simulink model "rhomodel"  (R2020a)
settings: Solver=VariableStepAuto  StartTime=0.0  StopTime=10.0  RelTol=1e-3
settings Model: Creator=marce  LastModifiedBy=marce

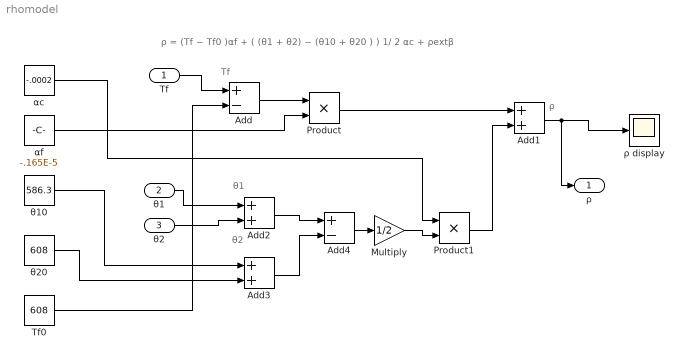
== system rhomodel ==
  note: Tf
  note: θ2
  note: θ1
  note: ρ
  note: ρ = (Tf − Tf0 )αf + ( (θ1 + θ2) − (θ10 + θ20 ) ) 1/ 2 αc + ρextβ
  Tf : Inport
  θ1 : Inport  Port=2
  θ2 : Inport  Port=3
  Add : Sum  Inputs=+-
  Add1 : Sum
  Add2 : Sum
  Add3 : Sum
  Add4 : Sum  Inputs=+-
  Multiply : Gain  Gain=1/2
  Product : Product
  Product1 : Product
  Tf0 : Constant  Value=608
  αc : Constant  Value=-.0002
  αf : Constant  Value=-.165E-5
  "θ10 " : Constant  Value=586.3
  θ20 : Constant  Value=608
  ρ display : Scope
  ρ : Outport
  wires:
  Add/1 -> Product/1
  Multiply/1 -> Product1/2
  Add3/1 -> Add4/2
  αc/1 -> Product1/1
  Add1/1 -> ρ/1, ρ display/1
  "θ10 "/1 -> Add3/1
  Add4/1 -> Multiply/1
  αf/1 -> Product/2
  Product/1 -> Add1/1
  Add2/1 -> Add4/1
  Tf0/1 -> Add/2
  θ20/1 -> Add3/2
  Product1/1 -> Add1/2
  θ1/1 -> Add2/1
  θ2/1 -> Add2/2
  Tf/1 -> Add/1
